simulink model "planGlobalPath"  (R2024a)
settings: Solver=FixedStepAuto  StartTime=0.0  StopTime=10.0  RelTol=1e-3
undefined symbols (not defined in the file or in its folder): maxRefPathLen
settings Model: Creator=cstabile  LastModifiedBy=cstabile
settings SFSimCC: SimTargetLang=C++

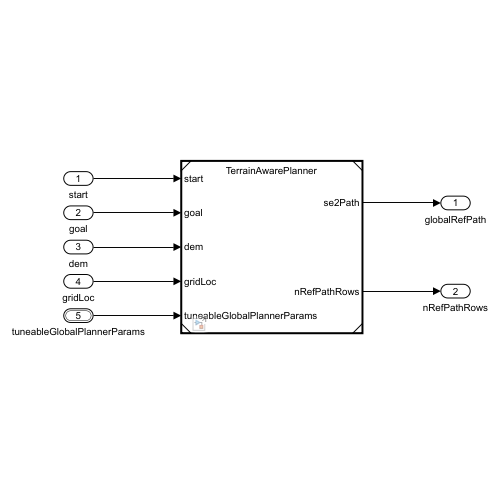
[thumbnail: Simulink's stored preview of the top-level diagram]
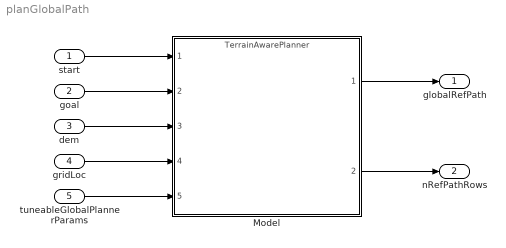
== system planGlobalPath ==
  start : Inport
  goal : Inport  Port=2
  dem : Inport  Port=3
  gridLoc : Inport  Port=4
  tuneableGlobalPlannerParams : Inport  Port=5  OutDataTypeStr=Bus: fsp_tunable_bus
  Model : ModelReference  ModelNameDialog=TerrainAwarePlanner.slx  SimulationMode=Normal  ModelReferenceVersion=2.0
  globalRefPath : Outport  PortDimensions=[maxRefPathLen 3]
  nRefPathRows : Outport  Port=2
  wires:
  gridLoc/1 -> Model/4
  dem/1 -> Model/3
  tuneableGlobalPlannerParams/1 -> Model/5
  Model/1 -> globalRefPath/1
  Model/2 -> nRefPathRows/1
  goal/1 -> Model/2
  start/1 -> Model/1
